simulink model "temp_1"  (Simulink 4.00)
settings: Solver=ode45  StartTime=0.0  StopTime=20000  MaxStep=1  RelTol=1e-3
values from neighbouring files (symbols this model uses):
  Ts = 0.5    [anfangsbed1.m]    (also in control_ident2.m; control_ident3.m; control_ident31.m; delay_1.m)
libraries: simulink3 x1
settings Model: LastModifiedBy=Administrator  BlockReductionOpt=off

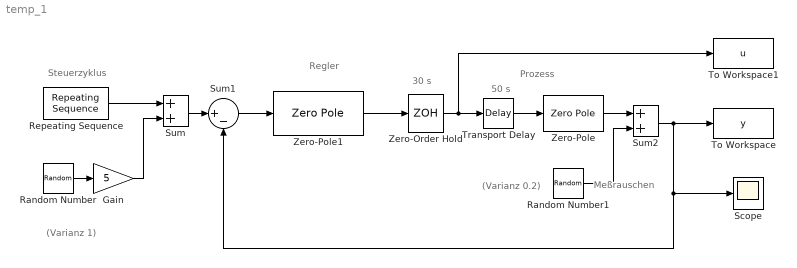
== system temp_1 ==
  note: (Varianz 0.2)
  note: (Varianz 1)
  note: Prozess
  note: Regler
  note: Meßrauschen
  note: Steuerzyklus
  note: 50 s
  note: 30 s
  Gain : Gain  Gain=5  Multiplication=Element-wise(K.*u)  SaturateOnIntegerOverflow=on
  Random Number : RandomNumber  Mean=0  Variance=1  Seed=12567  SampleTime=0
  Random Number1 : RandomNumber  Mean=0  Variance=0.2  Seed=79251  SampleTime=0
  Repeating Sequence : simulink3/Sources/Repeating Sequence  rep_seq_t=[0, 1800, 6000, 9000, 15000, 20000]  rep_seq_y=[0 200 200 500 500 0]
  Scope : Scope
      settings: TimeRange=30000  YMin=-100  YMax=800  SaveToWorkspace=off  SaveName=ScopeData  MaxDataPoints=5000
  Sum : Sum  Inputs=++  SaturateOnIntegerOverflow=on
  Sum1 : Sum  Inputs=|+-  SaturateOnIntegerOverflow=on
  Sum2 : Sum  Inputs=++  SaturateOnIntegerOverflow=on
  To Workspace : ToWorkspace  VariableName=y  SampleTime=Ts  SaveFormat=Array
  To Workspace1 : ToWorkspace  VariableName=u  SampleTime=Ts  SaveFormat=Array
  Transport Delay : TransportDelay  DelayTime=50  InitialInput=0  BufferSize=2048  PadeOrder=0
  Zero-Order Hold : ZeroOrderHold  SampleTime=30
  Zero-Pole : ZeroPole  Zeros=[]  Poles=[-0.0020]  Gain=[1]  AbsoluteTolerance=auto
  Zero-Pole1 : ZeroPole  Zeros=[ -0.002]  Poles=[0]  Gain=[0.01]  AbsoluteTolerance=auto
  wires:
  Random Number/1 -> Gain/1
  Repeating Sequence/1 -> Sum/1
  Gain/1 -> Sum/2
  Sum/1 -> Sum1/1
  Sum1/1 -> Zero-Pole1/1
  Zero-Pole1/1 -> Zero-Order Hold/1
  Zero-Order Hold/1 -> Transport Delay/1, To Workspace1/1
  Transport Delay/1 -> Zero-Pole/1
  Zero-Pole/1 -> Sum2/1
  Random Number1/1 -> Sum2/2
  Sum2/1 -> To Workspace/1, Sum1/2, Scope/1
